simulink model "fcn_1"  (Simulink 4.00)
settings: Solver=ode45  SolverMode=SingleTasking  StartTime=0.0  StopTime=10.0  FixedStep=0.1  RelTol=1e-3  AbsTol=1e-6
settings Model: LastModifiedBy=Administrator  ExtModeTrigMode=oneshot  ExtModeArmWhenConnect=off  BlockReductionOpt=off

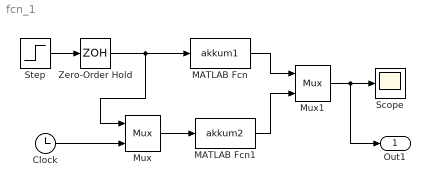
== system fcn_1 ==
  Clock : Clock
      settings: DisplayTime=off  Decimation=10
  MATLAB Fcn : MATLABFcn  MATLABFcn=akkum1  OutputDimensions=1  OutputSignalType=auto  Output1D=on
  MATLAB Fcn1 : MATLABFcn  MATLABFcn=akkum2  OutputDimensions=1  OutputSignalType=auto  Output1D=on
  Mux : Mux  Inputs=2
      settings: DisplayOption=none
  Mux1 : Mux  Inputs=2
      settings: DisplayOption=none
  Scope : Scope
      settings: TickLabels=on  TimeRange=auto  YMin=-5  YMax=300  SaveToWorkspace=off  SaveName=ScopeData  DataFormat=Array  LimitDataPoints=on  MaxDataPoints=5000
  Step : Step  Time=0  Before=0  After=1  SampleTime=0
  Zero-Order Hold : ZeroOrderHold  SampleTime=1
  Out1 : Outport  Port=1
  wires:
  MATLAB Fcn/1 -> Mux1/1
  Step/1 -> Zero-Order Hold/1
  Zero-Order Hold/1 -> MATLAB Fcn/1, Mux/1
  Mux1/1 -> Scope/1, Out1/1
  Clock/1 -> Mux/2
  Mux/1 -> MATLAB Fcn1/1
  MATLAB Fcn1/1 -> Mux1/2
